simulink model "model"  (R2021a)
settings: Solver=VariableStepAuto  StartTime=0.0  StopTime=20  FixedStep=1/2000  RelTol=1e-3
undefined symbols (not defined in the file or in its folder): DiscIntNeverNeededParam, F, F_I, g, K_lqr, Kf, L, l_p, l_rod, l_t, Local, m_c, m_p, m_wa, PendController, saturationVal, sys_ss, Ts, X, Y, Z
libraries: sm_lib x38, nesl_utility x8, pid_lib x4, sm_cable_examples_lib x4, simulink x2
(part 1 of 2)
settings Model: Creator=tmp  LastModifiedBy=jonas
settings DebuggingCC: SFMachineParentedDataDiag=warning

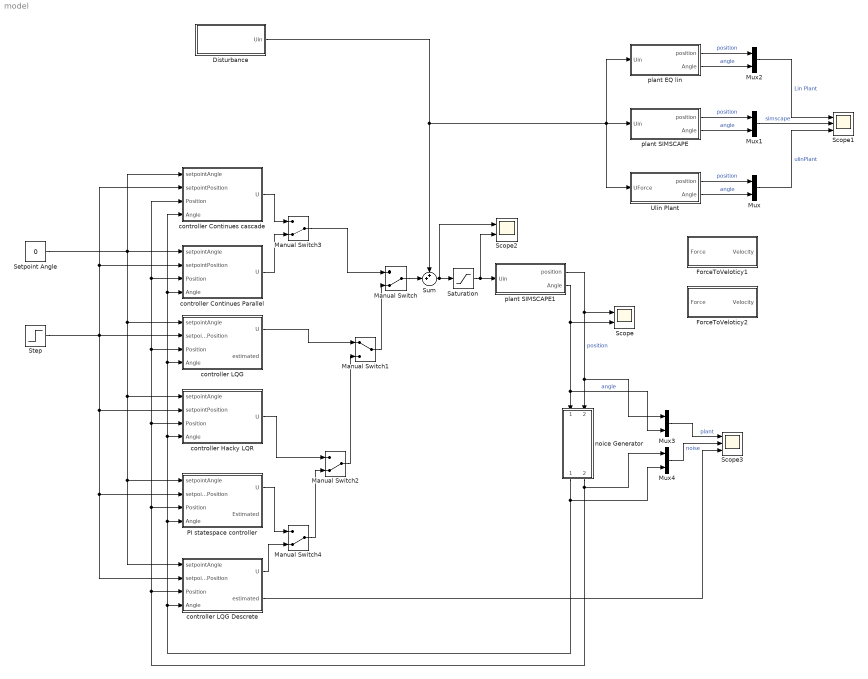
== system model ==
  Disturbance : Subsystem
  ForceToVeloticy1 : Subsystem
  ForceToVeloticy2 : Subsystem
  Manual Switch{,2..4} (4 alike) : ManualSwitch  CurrentSetting=0
  Manual Switch1 : ManualSwitch
  Mux{,1..4} (5 alike) : Mux  Inputs=2
  PI statespace controller : Subsystem
  Saturation : Saturate  UpperLimit=saturationVal  LowerLimit=-saturationVal
  Scope : Scope  NumInputPorts=2
  Scope1 : Scope  NumInputPorts=3
  Scope2 : Scope  NumInputPorts=2
  Scope3 : Scope  NumInputPorts=3
  Setpoint Angle : Constant  Value=0
  Step : Step  Time=5  After=0.5  SampleTime=0
  Sum : Sum  Inputs=++|
  Ulin Plant : Subsystem
  controller Continues Parallel : Subsystem
  controller Continues cascade : Subsystem
  controller Hacky LQR : Subsystem
  controller LQG : Subsystem
  controller LQG Descrete : Subsystem
  noice Generator : Subsystem
  plant EQ lin : Subsystem
  plant SIMSCAPE : Subsystem
  plant SIMSCAPE1 : Subsystem
  wires:
  plant SIMSCAPE1/1(position) -> Mux3/1, noice Generator/2(position), Scope/1  "position"
  plant SIMSCAPE1/2(Angle) -> Mux3/2, noice Generator/1(angle), Scope/2  "angle"
  Step/1 -> controller LQG Descrete/2(setpointPosition), PI statespace controller/2(setpointPosition), controller Hacky LQR/2(setpointPosition), controller LQG/2(setpointPosition), controller Continues cascade/2(setpointPosition), controller Continues Parallel/2(setpointPosition)
  Setpoint Angle/1 -> controller Continues cascade/1(setpointAngle), controller LQG/1(setpointAngle), controller LQG Descrete/1(setpointAngle), PI statespace controller/1(setpointAngle), controller Hacky LQR/1(setpointAngle), controller Continues Parallel/1(setpointAngle)
  Manual Switch3/1 -> Manual Switch/1
  controller Continues Parallel/1(U) -> Manual Switch3/2
  controller Continues cascade/1(U) -> Manual Switch3/1
  Sum/1 -> Saturation/1, Scope2/1
  Ulin Plant/1(position) -> Mux/1  "position"
  Ulin Plant/2(Angle) -> Mux/2  "angle"
  plant SIMSCAPE/1(position) -> Mux1/1  "position"
  plant SIMSCAPE/2(Angle) -> Mux1/2  "angle"
  Mux/1 -> Scope1/3  "ulinPlant"
  Mux1/1 -> Scope1/2  "simscape"
  Disturbance/1(Uin) -> Sum/1, Ulin Plant/1(UForce), plant EQ lin/1(Uin), plant SIMSCAPE/1(Uin)
  Manual Switch/1 -> Sum/2
  plant EQ lin/2(Angle) -> Mux2/2  "angle"
  plant EQ lin/1(position) -> Mux2/1  "position"
  Mux2/1 -> Scope1/1  "Lin Plant"
  controller LQG/1(U) -> Manual Switch1/1
  Manual Switch1/1 -> Manual Switch/2
  Manual Switch2/1 -> Manual Switch1/2
  controller Hacky LQR/1(U) -> Manual Switch2/1
  noice Generator/1(angleOut) -> Mux4/2, controller LQG Descrete/4(Angle), controller Continues cascade/4(Angle), controller Continues Parallel/4(Angle), controller LQG/4(Angle), controller Hacky LQR/4(Angle), PI statespace controller/4(Angle)
  noice Generator/2(positionOut) -> Mux4/1, controller Continues cascade/3(Position), controller Continues Parallel/3(Position), controller LQG/3(Position), controller Hacky LQR/3(Position), PI statespace controller/3(Position), controller LQG Descrete/3(Position)
  Mux3/1 -> Scope3/1  "plant"
  Mux4/1 -> Scope3/2  "noise"
  Saturation/1 -> plant SIMSCAPE1/1(Uin), Scope2/2
  controller LQG Descrete/1(U) -> Manual Switch4/2
  PI statespace controller/1(U) -> Manual Switch4/1
  Manual Switch4/1 -> Manual Switch2/2
  controller LQG Descrete/2(estimated) -> Scope3/3

== system model/Disturbance ==
  Gain1 : Gain
  Step2 : Step  SampleTime=0
  Step3 : Step  Time=1.1  After=-1  SampleTime=0
  Step4 : Step  Time=4  After=-0.5  SampleTime=0
  Step5 : Step  Time=4.1  After=0.5  SampleTime=0
  Sum3 : Sum  Inputs=++++
  Uin : Outport
  wires:
  Step5/1 -> Sum3/4
  Sum3/1 -> Gain1/1
  Step4/1 -> Sum3/3
  Gain1/1 -> Uin/1
  Step3/1 -> Sum3/2
  Step2/1 -> Sum3/1

== system model/ForceToVeloticy1 ==
  Force : Inport
  Gain : Gain  Gain=1/m_c
  Integrator : Integrator
  Velocity : Outport
  wires:
  Force/1 -> Gain/1
  Gain/1 -> Integrator/1
  Integrator/1 -> Velocity/1

== system model/ForceToVeloticy2 ==
  Force : Inport
  Gain : Gain  Gain=1/m_c
  Integrator : Integrator
  Velocity : Outport
  wires:
  Force/1 -> Gain/1
  Gain/1 -> Integrator/1
  Integrator/1 -> Velocity/1

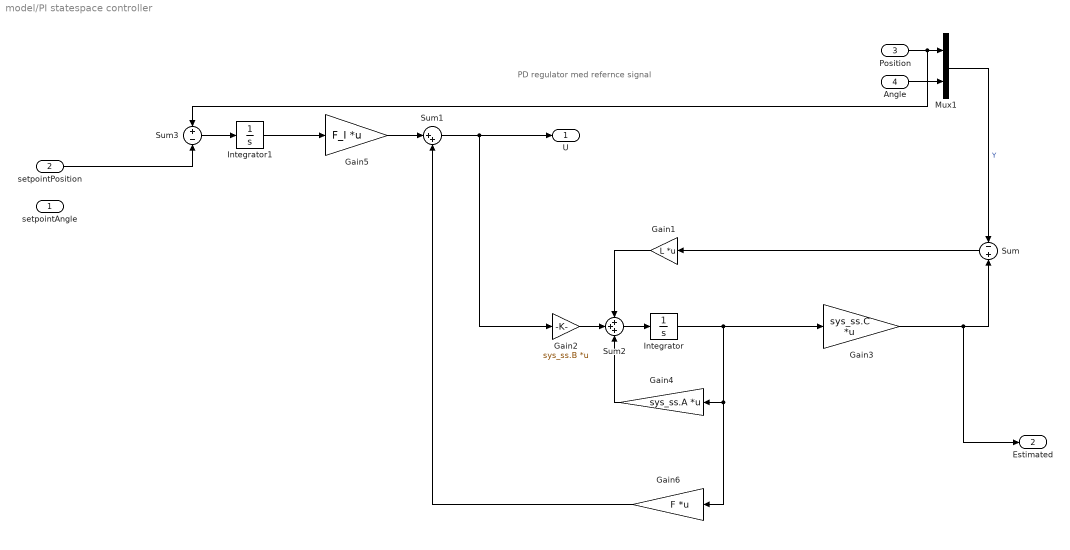
== system model/PI statespace controller ==
  note: PD regulator med refernce signal
  setpointAngle : Inport
  setpointPosition : Inport  Port=2
  Position : Inport  Port=3
  Angle : Inport  Port=4
  Gain1 : Gain  Gain=L  Multiplication=Matrix(K*u)
  Gain2 : Gain  Gain=sys_ss.B  Multiplication=Matrix(K*u)
  Gain3 : Gain  Gain=sys_ss.C  Multiplication=Matrix(K*u)
  Gain4 : Gain  Gain=sys_ss.A  Multiplication=Matrix(K*u)
  Gain5 : Gain  Gain=F_I  Multiplication=Matrix(K*u)
  Gain6 : Gain  Gain=F  Multiplication=Matrix(K*u)
  Integrator : Integrator  IgnoreLimit=on
  Integrator1 : Integrator
  Mux1 : Mux  Inputs=2
  Sum : Sum  Inputs=-+
  Sum1 : Sum  Inputs=|++
  Sum2 : Sum  Inputs=+++
  Sum3 : Sum  Inputs=+-
  U : Outport
  Estimated : Outport  Port=2
  wires:
  Angle/1 -> Mux1/2
  Position/1 -> Sum3/1, Mux1/1
  Gain1/1 -> Sum2/1
  Gain2/1 -> Sum2/2
  Gain3/1 -> Estimated/1, Sum/2
  Integrator/1 -> Gain6/1, Gain4/1, Gain3/1
  Gain4/1 -> Sum2/3
  Sum2/1 -> Integrator/1
  Sum/1 -> Gain1/1
  Mux1/1 -> Sum/1  "Y"
  Sum1/1 -> Gain2/1, U/1
  Gain5/1 -> Sum1/1
  Integrator1/1 -> Gain5/1
  Sum3/1 -> Integrator1/1
  Gain6/1 -> Sum1/2
  setpointPosition/1 -> Sum3/2

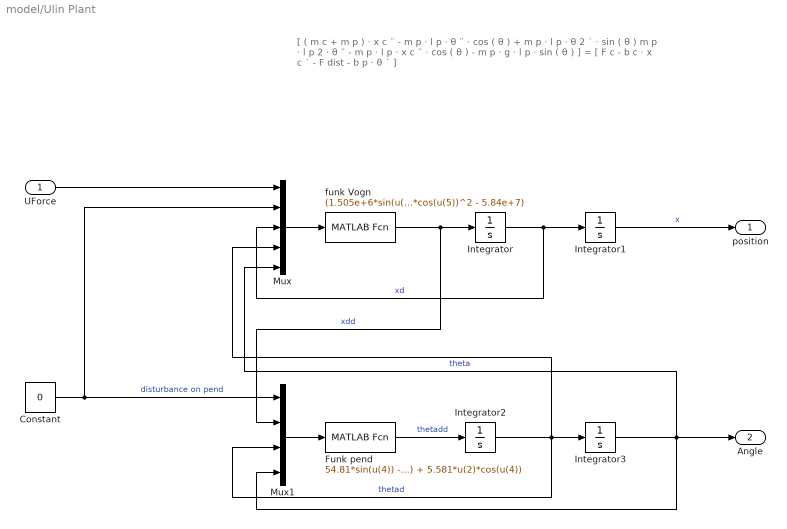
== system model/Ulin Plant ==
  note: [ ( m c + m p ) ⋅ x c ¨ - m p ⋅ l p ⋅ θ ¨ ⋅ cos ( θ ) + m p ⋅ l p ⋅ θ 2 ˙ ⋅ sin ( θ ) m p ⋅ l p 2 ⋅ θ ¨ - m p ⋅ l p ⋅ x c ¨ ⋅ cos ( θ ) - m p ⋅ g ⋅ l p ⋅ sin ( θ ) ] = [ F c - b c ⋅ x c ˙ - F dist - b p ⋅ θ ˙ ]
  UForce : Inport
  Constant : Constant  Value=0
  Funk pend : MATLABFcn  MATLABFcn=54.81*sin(u(4)) - 0.445*u(3) - 370.9*u(1) + 5.581*u(2)*cos(u(4))  OutputDimensions=1  Output1D=off
  Integrator{,1..3} (4 alike) : Integrator
  Mux : Mux  Inputs=5
  Mux1 : Mux
  funk Vogn : MATLABFcn  MATLABFcn=(1.505e+6*sin(u(5))*u(4)^2 + 6.697e+5*cos(u(5))*u(4) - 1.0e+8*u(1) + 5.0e+8*u(3) - 8.249e+7*cos(u(5))*sin(u(5)) + 5.582e+8*u(2)*cos(u(5)))/(8.4e+6*cos(u(5))^2 - 5.84e+7)  OutputDimensions=1  Output1D=off
  position : Outport
  Angle : Outport  Port=2
  wires:
  funk Vogn/1 -> Mux1/2, Integrator/1  "xdd"
  Mux/1 -> funk Vogn/1
  Integrator/1 -> Mux/3, Integrator1/1  "xd"
  Integrator1/1 -> position/1  "x"
  Integrator2/1 -> Mux/4, Mux1/3, Integrator3/1  "thetad"
  Funk pend/1 -> Integrator2/1  "thetadd"
  Mux1/1 -> Funk pend/1
  Integrator3/1 -> Mux/5, Mux1/4, Angle/1  "theta"
  UForce/1 -> Mux/1
  Constant/1 -> Mux1/1, Mux/2  "disturbance on pend"

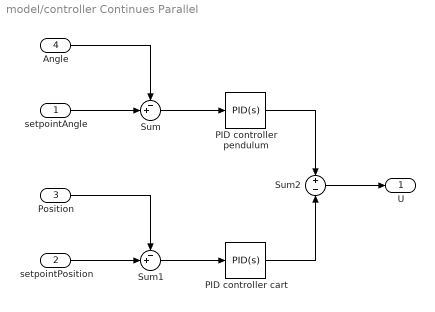
== system model/controller Continues Parallel ==
  setpointAngle : Inport
  setpointPosition : Inport  Port=2
  Position : Inport  Port=3
  Angle : Inport  Port=4
  PID controller cart : pid_lib/PID Controller  Controller=PID  Form=Parallel  TimeDomain=Continuous-time  UseExternalTs=off  SampleTime=-1  IntegratorMethod=Trapezoidal  FilterMethod=Forward Euler  ControllerParametersSource=internal  P=288.854597591641  I=22.5795684687671  D=-65.7392485263013  UseFilter=on  N=4.39394431891132  TunerSelectOption=Transfer Function Based (PID Tuner App)  InitialConditionSource=internal  InitialConditionForIntegrator=0  InitialConditionForFilter=0  DifferentiatorICPrevScaledInput=0  ExternalReset=none  TrackingMode=off  Kt=1  LimitOutput=off  SatLimitsSource=internal  UpperSaturationLimit=inf  LowerSaturationLimit=-inf  LinearizeAsGain=on  AntiWindupMode=none  Kb=1  POutMin=[]  POutMax=[]  IOutMin=[]  IOutMax=[]  DOutMin=[]  DOutMax=[]  NOutMin=[]  NOutMax=[]  SumOutMin=[]  SumOutMax=[]  SaturationOutMin=[]  SaturationOutMax=[]  PParamMin=[]  PParamMax=[]  IParamMin=[]  IParamMax=[]  DParamMin=[]  DParamMax=[]  NParamMin=[]  NParamMax=[]  KbParamMin=[]  KbParamMax=[]  KtParamMin=[]  KtParamMax=[]  KbOutMin=[]  KbOutMax=[]  KtOutMin=[]  KtOutMax=[]  IntegratorOutMin=[]  IntegratorOutMax=[]  FilterOutMin=[]  FilterOutMax=[]  SumI1OutMin=[]  SumI1OutMax=[]  SumI2OutMin=[]  SumI2OutMax=[]  SumI3OutMin=[]  SumI3OutMax=[]  SumI4OutMin=[]  SumI4OutMax=[]  SumDOutMin=[]  SumDOutMax=[]  DifferentiatorOutMin=[]  DifferentiatorOutMax=[]  FilterDiffOutCoefMin=[]  FilterDiffOutCoefMax=[]  ReciprocalOutMin=[]  ReciprocalOutMax=[]  SumDenOutMin=[]  SumDenOutMax=[]  SumNumOutMin=[]  SumNumOutMax=[]  DivideOutMin=[]  DivideOutMax=[]  UdiffTsProdOutMin=[]  UdiffTsProdOutMax=[]  NTsProdOutMin=[]  NTsProdOutMax=[]  UintegralTsProdOutMin=[]  UintegralTsProdOutMax=[]  UngainTsProdOutMin=[]  UngainTsProdOutMax=[]  IntegratorContinuousStateAttributes=''  IntegratorStateMustResolveToSignalObject=off  IntegratorRTWStateStorageClass=Auto  FilterContinuousStateAttributes=''  FilterStateMustResolveToSignalObject=off  FilterRTWStateStorageClass=Auto  ParallelPVariant=InternalParameters  IdealPVariant=Disabled  IVariant=InternalParameters  DVariant=InternalParameters  IntegratorVariant=Continuous  SatVariant=Disabled  AWVariant=Passthrough  PCopyVariant=Disabled  TRVariant=Disabled  FdbkBlocksVariant=Forward  IdealPFdbkVariant=Disabled  SatFdbkVariant=Disabled  DerivativeFilterVariant=ContFilter  NVariant=InternalParameters  NCopyVariant=Disabled  FilterICVariant=InternalICsFilter  IntegratorICVariant=InternalICs  ExternalResetVariant=Disabled  TRSumVariant=Passthrough  SumFdbkVariant=Disabled  SumVariant=Sum_PID  TsampFilterVariant=InternalTs  TsampNgainVariant=Passthrough  TsampIntegralVariant=Passthrough  ExternalSaturationOutDataTypeStr=Inherit: Same as second input
  PID controller pendulum : pid_lib/PID Controller  Controller=PID  Form=Parallel  TimeDomain=Continuous-time  UseExternalTs=off  SampleTime=-1  IntegratorMethod=Trapezoidal  FilterMethod=Trapezoidal  ControllerParametersSource=internal  P=PendController.Kp  I=PendController.Ki  D=PendController.Kd  UseFilter=on  N=PendController.Tf  TunerSelectOption=Transfer Function Based (PID Tuner App)  InitialConditionSource=internal  InitialConditionForIntegrator=0  InitialConditionForFilter=0  DifferentiatorICPrevScaledInput=0  ExternalReset=none  TrackingMode=off  Kt=1  LimitOutput=off  SatLimitsSource=internal  UpperSaturationLimit=inf  LowerSaturationLimit=-inf  LinearizeAsGain=on  AntiWindupMode=none  Kb=1  POutMin=[]  POutMax=[]  IOutMin=[]  IOutMax=[]  DOutMin=[]  DOutMax=[]  NOutMin=[]  NOutMax=[]  SumOutMin=[]  SumOutMax=[]  SaturationOutMin=[]  SaturationOutMax=[]  PParamMin=[]  PParamMax=[]  IParamMin=[]  IParamMax=[]  DParamMin=[]  DParamMax=[]  NParamMin=[]  NParamMax=[]  KbParamMin=[]  KbParamMax=[]  KtParamMin=[]  KtParamMax=[]  KbOutMin=[]  KbOutMax=[]  KtOutMin=[]  KtOutMax=[]  IntegratorOutMin=[]  IntegratorOutMax=[]  FilterOutMin=[]  FilterOutMax=[]  SumI1OutMin=[]  SumI1OutMax=[]  SumI2OutMin=[]  SumI2OutMax=[]  SumI3OutMin=[]  SumI3OutMax=[]  SumI4OutMin=[]  SumI4OutMax=[]  SumDOutMin=[]  SumDOutMax=[]  DifferentiatorOutMin=[]  DifferentiatorOutMax=[]  FilterDiffOutCoefMin=[]  FilterDiffOutCoefMax=[]  ReciprocalOutMin=[]  ReciprocalOutMax=[]  SumDenOutMin=[]  SumDenOutMax=[]  SumNumOutMin=[]  SumNumOutMax=[]  DivideOutMin=[]  DivideOutMax=[]  UdiffTsProdOutMin=[]  UdiffTsProdOutMax=[]  NTsProdOutMin=[]  NTsProdOutMax=[]  UintegralTsProdOutMin=[]  UintegralTsProdOutMax=[]  UngainTsProdOutMin=[]  UngainTsProdOutMax=[]  IntegratorContinuousStateAttributes=''  IntegratorStateMustResolveToSignalObject=off  IntegratorRTWStateStorageClass=Auto  FilterContinuousStateAttributes=''  FilterStateMustResolveToSignalObject=off  FilterRTWStateStorageClass=Auto  ParallelPVariant=InternalParameters  IdealPVariant=Disabled  IVariant=InternalParameters  DVariant=InternalParameters  IntegratorVariant=Continuous  SatVariant=Disabled  AWVariant=Passthrough  PCopyVariant=Disabled  TRVariant=Disabled  FdbkBlocksVariant=Forward  IdealPFdbkVariant=Disabled  SatFdbkVariant=Disabled  DerivativeFilterVariant=ContFilter  NVariant=InternalParameters  NCopyVariant=Disabled  FilterICVariant=InternalICsFilter  IntegratorICVariant=InternalICs  ExternalResetVariant=Disabled  TRSumVariant=Passthrough  SumFdbkVariant=Disabled  SumVariant=Sum_PID  TsampFilterVariant=InternalTs  TsampNgainVariant=Passthrough  TsampIntegralVariant=Passthrough  ExternalSaturationOutDataTypeStr=Inherit: Same as second input
  Sum : Sum  Inputs=-+|
  Sum1 : Sum  Inputs=-+|
  Sum2 : Sum  Inputs=+-
  U : Outport
  wires:
  setpointAngle/1 -> Sum/2
  setpointPosition/1 -> Sum1/2
  Sum1/1 -> PID controller cart/1
  Angle/1 -> Sum/1
  Position/1 -> Sum1/1
  Sum2/1 -> U/1
  PID controller pendulum/1 -> Sum2/1
  Sum/1 -> PID controller pendulum/1
  PID controller cart/1 -> Sum2/2

== system model/controller Continues cascade ==
  setpointAngle : Inport
  setpointPosition : Inport  Port=2
  Position : Inport  Port=3
  Angle : Inport  Port=4
  PID controller cart : pid_lib/PID Controller  Controller=PID  Form=Parallel  TimeDomain=Continuous-time  UseExternalTs=off  SampleTime=-1  IntegratorMethod=Trapezoidal  FilterMethod=Forward Euler  ControllerParametersSource=internal  P=-0.000734383045978884  I=-1.95673604455145e-06  D=-0.0382887909261764  UseFilter=on  N=0.989806605756417  TunerSelectOption=Transfer Function Based (PID Tuner App)  InitialConditionSource=internal  InitialConditionForIntegrator=0  InitialConditionForFilter=0  DifferentiatorICPrevScaledInput=0  ExternalReset=none  TrackingMode=off  Kt=1  LimitOutput=off  SatLimitsSource=internal  UpperSaturationLimit=inf  LowerSaturationLimit=-inf  LinearizeAsGain=on  AntiWindupMode=none  Kb=1  POutMin=[]  POutMax=[]  IOutMin=[]  IOutMax=[]  DOutMin=[]  DOutMax=[]  NOutMin=[]  NOutMax=[]  SumOutMin=[]  SumOutMax=[]  SaturationOutMin=[]  SaturationOutMax=[]  PParamMin=[]  PParamMax=[]  IParamMin=[]  IParamMax=[]  DParamMin=[]  DParamMax=[]  NParamMin=[]  NParamMax=[]  KbParamMin=[]  KbParamMax=[]  KtParamMin=[]  KtParamMax=[]  KbOutMin=[]  KbOutMax=[]  KtOutMin=[]  KtOutMax=[]  IntegratorOutMin=[]  IntegratorOutMax=[]  FilterOutMin=[]  FilterOutMax=[]  SumI1OutMin=[]  SumI1OutMax=[]  SumI2OutMin=[]  SumI2OutMax=[]  SumI3OutMin=[]  SumI3OutMax=[]  SumI4OutMin=[]  SumI4OutMax=[]  SumDOutMin=[]  SumDOutMax=[]  DifferentiatorOutMin=[]  DifferentiatorOutMax=[]  FilterDiffOutCoefMin=[]  FilterDiffOutCoefMax=[]  ReciprocalOutMin=[]  ReciprocalOutMax=[]  SumDenOutMin=[]  SumDenOutMax=[]  SumNumOutMin=[]  SumNumOutMax=[]  DivideOutMin=[]  DivideOutMax=[]  UdiffTsProdOutMin=[]  UdiffTsProdOutMax=[]  NTsProdOutMin=[]  NTsProdOutMax=[]  UintegralTsProdOutMin=[]  UintegralTsProdOutMax=[]  UngainTsProdOutMin=[]  UngainTsProdOutMax=[]  IntegratorContinuousStateAttributes=''  IntegratorStateMustResolveToSignalObject=off  IntegratorRTWStateStorageClass=Auto  FilterContinuousStateAttributes=''  FilterStateMustResolveToSignalObject=off  FilterRTWStateStorageClass=Auto  ParallelPVariant=InternalParameters  IdealPVariant=Disabled  IVariant=InternalParameters  DVariant=InternalParameters  IntegratorVariant=Continuous  SatVariant=Disabled  AWVariant=Passthrough  PCopyVariant=Disabled  TRVariant=Disabled  FdbkBlocksVariant=Forward  IdealPFdbkVariant=Disabled  SatFdbkVariant=Disabled  DerivativeFilterVariant=ContFilter  NVariant=InternalParameters  NCopyVariant=Disabled  FilterICVariant=InternalICsFilter  IntegratorICVariant=InternalICs  ExternalResetVariant=Disabled  TRSumVariant=Passthrough  SumFdbkVariant=Disabled  SumVariant=Sum_PID  TsampFilterVariant=InternalTs  TsampNgainVariant=Passthrough  TsampIntegralVariant=Passthrough  ExternalSaturationOutDataTypeStr=Inherit: Same as second input
  PID controller pendulum : pid_lib/PID Controller  Controller=PID  Form=Parallel  TimeDomain=Continuous-time  UseExternalTs=off  SampleTime=-1  IntegratorMethod=Trapezoidal  FilterMethod=Trapezoidal  ControllerParametersSource=internal  P=PendController.Kp  I=PendController.Ki  D=PendController.Kd  UseFilter=on  N=PendController.Tf  TunerSelectOption=Transfer Function Based (PID Tuner App)  InitialConditionSource=internal  InitialConditionForIntegrator=0  InitialConditionForFilter=0  DifferentiatorICPrevScaledInput=0  ExternalReset=none  TrackingMode=off  Kt=1  LimitOutput=off  SatLimitsSource=internal  UpperSaturationLimit=inf  LowerSaturationLimit=-inf  LinearizeAsGain=on  AntiWindupMode=none  Kb=1  POutMin=[]  POutMax=[]  IOutMin=[]  IOutMax=[]  DOutMin=[]  DOutMax=[]  NOutMin=[]  NOutMax=[]  SumOutMin=[]  SumOutMax=[]  SaturationOutMin=[]  SaturationOutMax=[]  PParamMin=[]  PParamMax=[]  IParamMin=[]  IParamMax=[]  DParamMin=[]  DParamMax=[]  NParamMin=[]  NParamMax=[]  KbParamMin=[]  KbParamMax=[]  KtParamMin=[]  KtParamMax=[]  KbOutMin=[]  KbOutMax=[]  KtOutMin=[]  KtOutMax=[]  IntegratorOutMin=[]  IntegratorOutMax=[]  FilterOutMin=[]  FilterOutMax=[]  SumI1OutMin=[]  SumI1OutMax=[]  SumI2OutMin=[]  SumI2OutMax=[]  SumI3OutMin=[]  SumI3OutMax=[]  SumI4OutMin=[]  SumI4OutMax=[]  SumDOutMin=[]  SumDOutMax=[]  DifferentiatorOutMin=[]  DifferentiatorOutMax=[]  FilterDiffOutCoefMin=[]  FilterDiffOutCoefMax=[]  ReciprocalOutMin=[]  ReciprocalOutMax=[]  SumDenOutMin=[]  SumDenOutMax=[]  SumNumOutMin=[]  SumNumOutMax=[]  DivideOutMin=[]  DivideOutMax=[]  UdiffTsProdOutMin=[]  UdiffTsProdOutMax=[]  NTsProdOutMin=[]  NTsProdOutMax=[]  UintegralTsProdOutMin=[]  UintegralTsProdOutMax=[]  UngainTsProdOutMin=[]  UngainTsProdOutMax=[]  IntegratorContinuousStateAttributes=''  IntegratorStateMustResolveToSignalObject=off  IntegratorRTWStateStorageClass=Auto  FilterContinuousStateAttributes=''  FilterStateMustResolveToSignalObject=off  FilterRTWStateStorageClass=Auto  ParallelPVariant=InternalParameters  IdealPVariant=Disabled  IVariant=InternalParameters  DVariant=InternalParameters  IntegratorVariant=Continuous  SatVariant=Disabled  AWVariant=Passthrough  PCopyVariant=Disabled  TRVariant=Disabled  FdbkBlocksVariant=Forward  IdealPFdbkVariant=Disabled  SatFdbkVariant=Disabled  DerivativeFilterVariant=ContFilter  NVariant=InternalParameters  NCopyVariant=Disabled  FilterICVariant=InternalICsFilter  IntegratorICVariant=InternalICs  ExternalResetVariant=Disabled  TRSumVariant=Passthrough  SumFdbkVariant=Disabled  SumVariant=Sum_PID  TsampFilterVariant=InternalTs  TsampNgainVariant=Passthrough  TsampIntegralVariant=Passthrough  ExternalSaturationOutDataTypeStr=Inherit: Same as second input
  Sum : Sum  Inputs=-+|
  Sum1 : Sum  Inputs=-+|
  U : Outport
  wires:
  setpointPosition/1 -> Sum1/2
  Sum1/1 -> PID controller cart/1
  Angle/1 -> Sum/1
  Position/1 -> Sum1/1
  PID controller pendulum/1 -> U/1
  Sum/1 -> PID controller pendulum/1
  PID controller cart/1 -> Sum/2

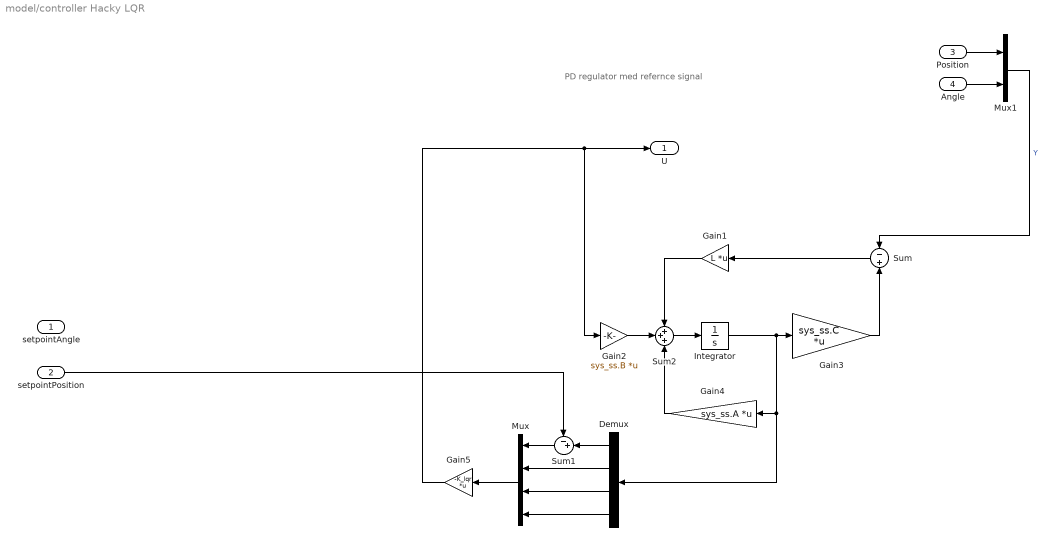
== system model/controller Hacky LQR ==
  note: PD regulator med refernce signal
  setpointAngle : Inport
  setpointPosition : Inport  Port=2
  Position : Inport  Port=3
  Angle : Inport  Port=4
  Demux : Demux
  Gain1 : Gain  Gain=L  Multiplication=Matrix(K*u)
  Gain2 : Gain  Gain=sys_ss.B  Multiplication=Matrix(K*u)
  Gain3 : Gain  Gain=sys_ss.C  Multiplication=Matrix(K*u)
  Gain4 : Gain  Gain=sys_ss.A  Multiplication=Matrix(K*u)
  Gain5 : Gain  Gain=-K_lqr  Multiplication=Matrix(K*u)
  Integrator : Integrator  IgnoreLimit=on
  Mux : Mux
  Mux1 : Mux  Inputs=2
  Sum : Sum  Inputs=-+
  Sum1 : Sum  Inputs=-+|
  Sum2 : Sum  Inputs=+++
  U : Outport
  wires:
  Angle/1 -> Mux1/2
  Position/1 -> Mux1/1
  Gain1/1 -> Sum2/1
  Gain2/1 -> Sum2/2
  Gain3/1 -> Sum/2
  Integrator/1 -> Demux/1, Gain4/1, Gain3/1
  Gain4/1 -> Sum2/3
  Sum2/1 -> Integrator/1
  Sum/1 -> Gain1/1
  Mux1/1 -> Sum/1  "Y"
  Mux/1 -> Gain5/1
  Demux/2 -> Mux/2
  Demux/3 -> Mux/3
  Demux/4 -> Mux/4
  Sum1/1 -> Mux/1
  Demux/1 -> Sum1/2
  setpointPosition/1 -> Sum1/1
  Gain5/1 -> Gain2/1, U/1

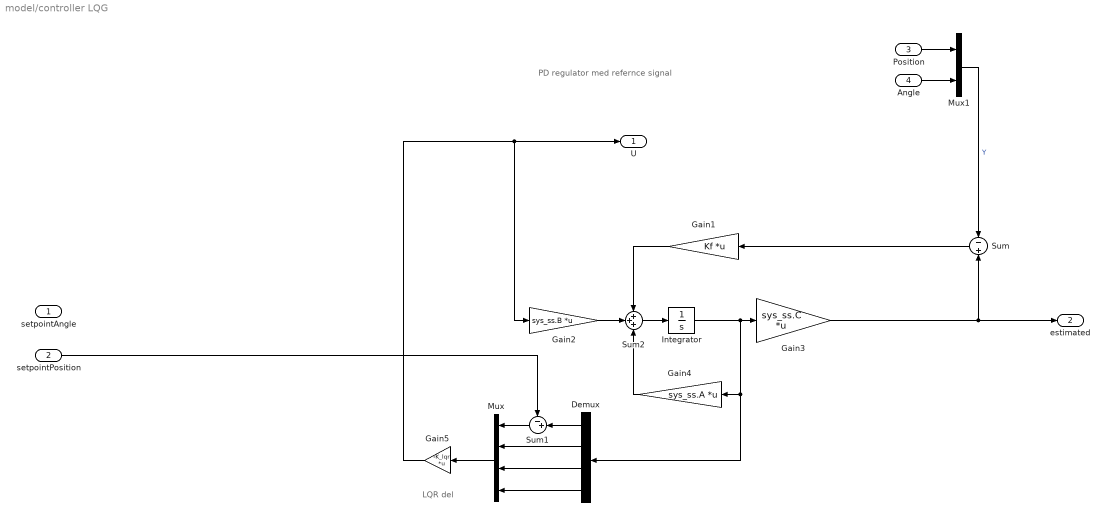
== system model/controller LQG ==
  note: LQR del
  note: PD regulator med refernce signal
  setpointAngle : Inport
  setpointPosition : Inport  Port=2
  Position : Inport  Port=3
  Angle : Inport  Port=4
  Demux : Demux
  Gain1 : Gain  Gain=Kf  Multiplication=Matrix(K*u)
  Gain2 : Gain  Gain=sys_ss.B  Multiplication=Matrix(K*u)
  Gain3 : Gain  Gain=sys_ss.C  Multiplication=Matrix(K*u)
  Gain4 : Gain  Gain=sys_ss.A  Multiplication=Matrix(K*u)
  Gain5 : Gain  Gain=-K_lqr  Multiplication=Matrix(K*u)
  Integrator : Integrator  IgnoreLimit=on
  Mux : Mux
  Mux1 : Mux  Inputs=2
  Sum : Sum  Inputs=-+
  Sum1 : Sum  Inputs=-+|
  Sum2 : Sum  Inputs=+++
  U : Outport
  estimated : Outport  Port=2
  wires:
  Angle/1 -> Mux1/2
  Position/1 -> Mux1/1
  Gain1/1 -> Sum2/1
  Gain2/1 -> Sum2/2
  Gain3/1 -> estimated/1, Sum/2
  Gain4/1 -> Sum2/3
  Sum2/1 -> Integrator/1
  Sum/1 -> Gain1/1
  Mux1/1 -> Sum/1  "Y"
  Mux/1 -> Gain5/1
  Demux/2 -> Mux/2
  Demux/3 -> Mux/3
  Demux/4 -> Mux/4
  Sum1/1 -> Mux/1
  Demux/1 -> Sum1/2
  setpointPosition/1 -> Sum1/1
  Gain5/1 -> U/1, Gain2/1
  Integrator/1 -> Demux/1, Gain4/1, Gain3/1

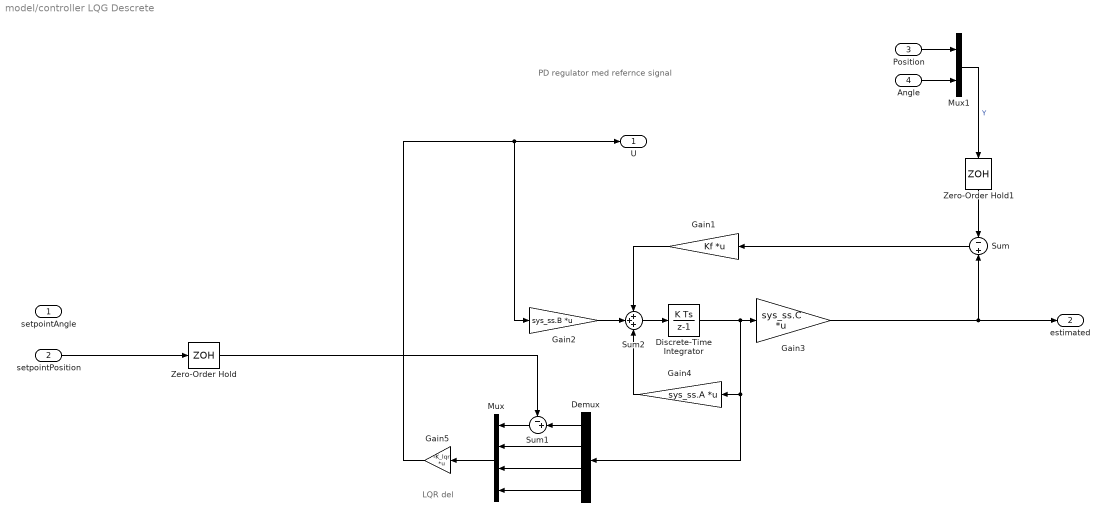
== system model/controller LQG Descrete ==
  note: LQR del
  note: PD regulator med refernce signal
  setpointAngle : Inport
  setpointPosition : Inport  Port=2
  Position : Inport  Port=3
  Angle : Inport  Port=4
  Demux : Demux
  Discrete-Time Integrator : DiscreteIntegrator  SampleTime=Ts  ICPrevOutput=DiscIntNeverNeededParam  ICPrevScaledInput=DiscIntNeverNeededParam
  Gain1 : Gain  Gain=Kf  Multiplication=Matrix(K*u)
  Gain2 : Gain  Gain=sys_ss.B  Multiplication=Matrix(K*u)
  Gain3 : Gain  Gain=sys_ss.C  Multiplication=Matrix(K*u)
  Gain4 : Gain  Gain=sys_ss.A  Multiplication=Matrix(K*u)
  Gain5 : Gain  Gain=-K_lqr  Multiplication=Matrix(K*u)
  Mux : Mux
  Mux1 : Mux  Inputs=2
  Sum : Sum  Inputs=-+
  Sum1 : Sum  Inputs=-+|
  Sum2 : Sum  Inputs=+++
  Zero-Order Hold : ZeroOrderHold  SampleTime=Ts
  Zero-Order Hold1 : ZeroOrderHold  SampleTime=Ts
  U : Outport
  estimated : Outport  Port=2
  wires:
  Angle/1 -> Mux1/2
  Position/1 -> Mux1/1
  Gain1/1 -> Sum2/1
  Gain2/1 -> Sum2/2
  Gain3/1 -> estimated/1, Sum/2
  Gain4/1 -> Sum2/3
  Sum2/1 -> Discrete-Time Integrator/1
  Sum/1 -> Gain1/1
  Mux1/1 -> Zero-Order Hold1/1  "Y"
  Mux/1 -> Gain5/1
  Demux/2 -> Mux/2
  Demux/3 -> Mux/3
  Demux/4 -> Mux/4
  Sum1/1 -> Mux/1
  Demux/1 -> Sum1/2
  setpointPosition/1 -> Zero-Order Hold/1
  Gain5/1 -> U/1, Gain2/1
  Discrete-Time Integrator/1 -> Demux/1, Gain4/1, Gain3/1
  Zero-Order Hold/1 -> Sum1/1
  Zero-Order Hold1/1 -> Sum/1

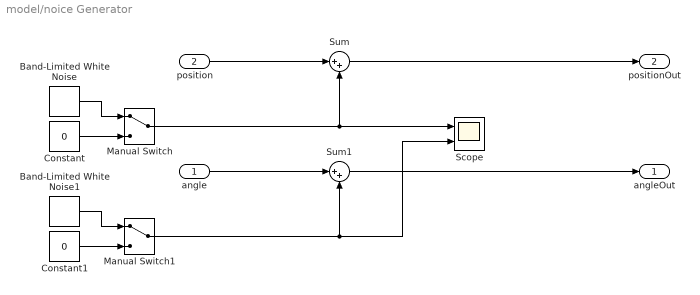
== system model/noice Generator ==
  angle : Inport
  position : Inport  Port=2
  Band-Limited White Noise : simulink/Sources/Band-Limited White Noise  Cov=[0.0000001]  Ts=0.01  seed=[23341]
  Band-Limited White Noise1 : simulink/Sources/Band-Limited White Noise  Cov=[0.0000001]  Ts=0.01  seed=[10000]
  Constant : Constant  Value=0
  Constant1 : Constant  Value=0
  Manual Switch : ManualSwitch
  Manual Switch1 : ManualSwitch
  Scope : Scope  NumInputPorts=2
  Sum : Sum  Inputs=|++
  Sum1 : Sum  Inputs=|++
  angleOut : Outport
  positionOut : Outport  Port=2
  wires:
  position/1 -> Sum/1
  Sum/1 -> positionOut/1
  Sum1/1 -> angleOut/1
  angle/1 -> Sum1/1
  Band-Limited White Noise/1 -> Manual Switch/1
  Constant/1 -> Manual Switch/2
  Constant1/1 -> Manual Switch1/2
  Band-Limited White Noise1/1 -> Manual Switch1/1
  Manual Switch1/1 -> Sum1/2, Scope/2
  Manual Switch/1 -> Sum/2, Scope/1

== system model/plant EQ lin ==
  Uin : Inport
  Demux : Demux
  State-Space : StateSpace  A=sys_ss.A  B=sys_ss.B  C=eye(4)  D=[0;0;0;0]  InitialCondition=0
  position : Outport
  Angle : Outport  Port=2
  wires:
  Uin/1 -> State-Space/1
  Demux/3 -> Angle/1
  State-Space/1 -> Demux/1
  Demux/1 -> position/1

== system model/plant SIMSCAPE ==
  Uin : Inport
  Base : Subsystem
  Configuration : Subsystem
  PS-Simulink Converter : nesl_utility/PS-Simulink Converter  PhysicalDomain=network_engine_domain  SubClassName=ps_output  LeftPortType=input  RightPortType=output  PseudoPeriodic=off  Frequencies=[]  Unit=inherit  AffineConversion=off
      settings: SourceProductBaseCode=PW,SS
  PS-Simulink Converter1 : nesl_utility/PS-Simulink Converter  PhysicalDomain=network_engine_domain  SubClassName=ps_output  LeftPortType=input  RightPortType=output  PseudoPeriodic=off  Frequencies=[]  Unit=inherit  AffineConversion=off
      settings: SourceProductBaseCode=PW,SS
  Plant : Subsystem
      settings: PortSchema="{\"entries\":[{\"content\":{\"sides\":[{\"content\":{\"connectorIds\":[\"LConn1\",\"In1\",\"LConn2\",\"LConn3\"]},\"type\":\"ConnectorPlacement.EquallySpacedRectSide\",\"uuid\":\"e241dd80-f9a1-4c3d-bd3c-4b3bd119c000\"},{\"content\":{\"connectorIds\":[],\"side\":\"RIGHT\"},\"type\":\"ConnectorPlacement.EquallySpacedRectSide\",\"uuid\":\"50ff246f-1c39-4ae1-b10f-6d3ede22cdb7\"},{\"content\":{\"connectorIds\":[],\"side\":\"TOP\"},\"type\":\"ConnectorPlacement.EquallySpacedRectSide\",\"uuid\":\"3277ae83-9f73-4616-bf6d-fc59e06ded2c\"}]},\"type\":\"ConnectorPlacement.EquallySpacedConnector\",\"uuid\":\"16b9ee55-2353-4e36-979f-af01577ad86e\"}],\"packageUris\":[\"http://schema.mathworks.com/mf0/Connector/R2020b\"],\"version\":\"1.0\"}"
  position : Outport
  Angle : Outport  Port=2
  wires:
  Uin/1 -> Plant/1(force)
  PS-Simulink Converter/1 -> position/1
  PS-Simulink Converter1/1 -> Angle/1
  connections:
  Base/RConn3 -- Configuration/RConn1 -- Plant/LConn1
  PS-Simulink Converter/LConn1 -- Plant/LConn3
  PS-Simulink Converter1/LConn1 -- Plant/LConn2

== system model/plant SIMSCAPE1 ==
  Uin : Inport
  Base : Subsystem
  Configuration : Subsystem
  PS-Simulink Converter : nesl_utility/PS-Simulink Converter  PhysicalDomain=network_engine_domain  SubClassName=ps_output  LeftPortType=input  RightPortType=output  PseudoPeriodic=off  Frequencies=[]  Unit=inherit  AffineConversion=off
      settings: SourceProductBaseCode=PW,SS
  PS-Simulink Converter1 : nesl_utility/PS-Simulink Converter  PhysicalDomain=network_engine_domain  SubClassName=ps_output  LeftPortType=input  RightPortType=output  PseudoPeriodic=off  Frequencies=[]  Unit=inherit  AffineConversion=off
      settings: SourceProductBaseCode=PW,SS
  Plant : Subsystem
      settings: PortSchema="{\"entries\":[{\"content\":{\"sides\":[{\"content\":{\"connectorIds\":[\"LConn1\",\"In1\",\"LConn2\",\"LConn3\"]},\"type\":\"ConnectorPlacement.EquallySpacedRectSide\",\"uuid\":\"e241dd80-f9a1-4c3d-bd3c-4b3bd119c000\"},{\"content\":{\"connectorIds\":[],\"side\":\"RIGHT\"},\"type\":\"ConnectorPlacement.EquallySpacedRectSide\",\"uuid\":\"50ff246f-1c39-4ae1-b10f-6d3ede22cdb7\"},{\"content\":{\"connectorIds\":[],\"side\":\"TOP\"},\"type\":\"ConnectorPlacement.EquallySpacedRectSide\",\"uuid\":\"3277ae83-9f73-4616-bf6d-fc59e06ded2c\"}]},\"type\":\"ConnectorPlacement.EquallySpacedConnector\",\"uuid\":\"16b9ee55-2353-4e36-979f-af01577ad86e\"}],\"packageUris\":[\"http://schema.mathworks.com/mf0/Connector/R2020b\"],\"version\":\"1.0\"}"
  position : Outport
  Angle : Outport  Port=2
  wires:
  Uin/1 -> Plant/1(force)
  PS-Simulink Converter/1 -> position/1
  PS-Simulink Converter1/1 -> Angle/1
  connections:
  Base/RConn3 -- Configuration/RConn1 -- Plant/LConn1
  PS-Simulink Converter/LConn1 -- Plant/LConn3
  PS-Simulink Converter1/LConn1 -- Plant/LConn2

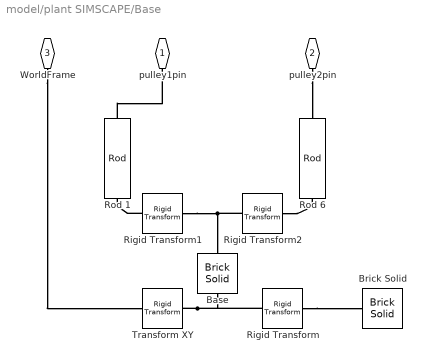
== system model/plant SIMSCAPE/Base ==
  Base : sm_lib/Body Elements/Brick Solid  GraphicAmbientColor=[0.15 0.15 0.15 1.0]  BasedOnType=Density  BrickDimensions=[l_t+0.1 0.02 0.1]  BrickDimensionUnits=m  CenterOfMass=[0 0 0]  CenterOfMassUnits=m  GraphicDiffuseColor=[1.0 1.0 1.0]  Density=1000  DensityUnits=kg/m^3  DoExposeReferenceFrame=off  GraphicEmissiveColor=[0.0 0.0 0.0 1.0]  ExportEntireGeometry=off  SerializedFrames=<Frames><Frame><Id>Frame1</Id><Value><Name>T</Name><Origin><Source>GeometricFeature</Source><FeatureName>+z surface</FeatureName></Origin><PrimaryAxis><DefinedDirection>+Z</DefinedDirection><Source>ReferenceFrame</Source><SourceDirection>+Z</SourceDirection><FeatureName></FeatureName></PrimaryAxis><SecondaryAxis><DefinedDirection>+X</DefinedDirection><Source>ReferenceFrame</Source><SourceDirection>+X</SourceDirection><FeatureName></FeatureName></SecondaryAxis></Value></Frame><Frame><Id>Frame2</Id><Value><Name>B</Name><Origin><Source>GeometricFeature</Source><FeatureName>-z surface</FeatureName></Origin><PrimaryAxis><DefinedDirection>+Z</DefinedDirection><Source>ReferenceFrame</Source><SourceDirection>+Z</SourceDirection><FeatureName></FeatureName></PrimaryAxis><SecondaryAxis><DefinedDirection>+X</DefinedDirection><Source>ReferenceFrame</Source><SourceDirection>+X</SourceDirection><FeatureName></FeatureName></SecondaryAxis></Value></Frame></Frames>  MarkerShape=Sphere  MarkerSize=10  GraphicType=FromGeometry  InertiaType=CalculateFromGeometry  Mass=1  MassUnits=kg  MomentsOfInertia=[1 1 1]  MomentsOfInertiaUnits=kg*m^2  GraphicOpacity=0.75  ProductsOfInertia=[0 0 0]  ProductsOfInertiaUnits=kg*m^2  GraphicShininess=128  GraphicSpecularColor=[0.5 0.5 0.5 1.0]  GraphicVisPropType=SimpleVisualProperties
      settings: SourceProductName=Multibody
  Brick Solid : sm_lib/Body Elements/Brick Solid  GraphicAmbientColor=[0.15 0.15 0.15 1.0]  BasedOnType=Density  BrickDimensions=[l_t 0.05 0.01]  BrickDimensionUnits=m  CenterOfMass=[0 0 0]  CenterOfMassUnits=m  GraphicDiffuseColor=[0.8 0.8 0.8]  Density=1000  DensityUnits=kg/m^3  DoExposeReferenceFrame=on  GraphicEmissiveColor=[0.0 0.0 0.0 1.0]  ExportEntireGeometry=off  SerializedFrames=<Frames/>  MarkerShape=Sphere  MarkerSize=10  GraphicType=FromGeometry  InertiaType=CalculateFromGeometry  Mass=1  MassUnits=kg  MomentsOfInertia=[1 1 1]  MomentsOfInertiaUnits=kg*m^2  GraphicOpacity=1.0  ProductsOfInertia=[0 0 0]  ProductsOfInertiaUnits=kg*m^2  GraphicShininess=75  GraphicSpecularColor=[0.5 0.5 0.5 1.0]  GraphicVisPropType=SimpleVisualProperties
  Rigid Transform : sm_lib/Frames and Transforms/Rigid Transform  TranslationMethod=Cartesian  TranslationStandardOffset=0  TranslationLengthUnit=m  TranslationStandardAxis=+Z  TranslationCartesianOffset=[0 -0.03 0.0825]  TranslationROffset=0  TranslationROffsetUnits=m  TranslationZOffset=0  TranslationZOffsetUnits=m  TranslationThetaOffset=0  TranslationThetaOffsetUnits=deg  RotationMethod=None  RotationAngleUnits=deg  RotationStandardAxis=+Z  RotationAngle=0.0  RotationArbitraryAxis=[0 0 1]  FollAlignAxisA=+X  BaseAlignAxisA=+Y  FollAlignAxisB=+Y  BaseAlignAxisB=+Z  RotationSequenceAxes=FollowerAxes  RotationSequence=XYX  RotationSequenceAngles=[0 0 0]  RotationSequenceAnglesUnits=deg  RotationMatrix=[1 0 0; 0 1 0; 0 0 1]
  Rigid Transform1 : sm_lib/Frames and Transforms/Rigid Transform  TranslationMethod=Cartesian  TranslationStandardOffset=0  TranslationLengthUnit=m  TranslationStandardAxis=+Z  TranslationCartesianOffset=[-l_t/2 0 -0.05]  TranslationROffset=0  TranslationROffsetUnits=m  TranslationZOffset=0  TranslationZOffsetUnits=m  TranslationThetaOffset=0  TranslationThetaOffsetUnits=deg  RotationMethod=StandardAxis  RotationAngleUnits=deg  RotationStandardAxis=+X  RotationAngle=90  RotationArbitraryAxis=[0 0 1]  FollAlignAxisA=+X  BaseAlignAxisA=+Y  FollAlignAxisB=+Y  BaseAlignAxisB=+Z  RotationSequenceAxes=FollowerAxes  RotationSequence=XYX  RotationSequenceAngles=[0 0 0]  RotationSequenceAnglesUnits=deg  RotationMatrix=[1 0 0; 0 1 0; 0 0 1]
  Rigid Transform2 : sm_lib/Frames and Transforms/Rigid Transform  TranslationMethod=Cartesian  TranslationStandardOffset=0  TranslationLengthUnit=m  TranslationStandardAxis=+Z  TranslationCartesianOffset=[l_t/2 0 -0.05]  TranslationROffset=0  TranslationROffsetUnits=m  TranslationZOffset=0  TranslationZOffsetUnits=m  TranslationThetaOffset=0  TranslationThetaOffsetUnits=deg  RotationMethod=StandardAxis  RotationAngleUnits=deg  RotationStandardAxis=+X  RotationAngle=90  RotationArbitraryAxis=[0 0 1]  FollAlignAxisA=+X  BaseAlignAxisA=+Y  FollAlignAxisB=+Y  BaseAlignAxisB=+Z  RotationSequenceAxes=FollowerAxes  RotationSequence=XYX  RotationSequenceAngles=[0 0 0]  RotationSequenceAnglesUnits=deg  RotationMatrix=[1 0 0; 0 1 0; 0 0 1]
  Rod 1 : sm_cable_examples_lib/Basic/Rod  rod_rad=0.01  rod_len=0.05  rod_rho=7000  rod_color=[0.5 0.5 0.5]  popup_zori=Local +Z  popup_markings=None  mark_radius_range=[0.5 1.01]  mark_length_range=1.005  mark_angle_range=30  mark_color=[1 1 1]
      link override Transform F: TranslationStandardOffset=rod_len/4*z_ori
      settings: SourceProductBaseCode=MS
  Rod 6 : sm_cable_examples_lib/Basic/Rod  rod_rad=0.01  rod_len=0.05  rod_rho=7000  rod_color=[0.5 0.5 0.5]  popup_zori=Local +Z  popup_markings=None  mark_radius_range=[0.5 1.01]  mark_length_range=1.005  mark_angle_range=30  mark_color=[1 1 1]
      link override Transform F: TranslationStandardOffset=rod_len/4*z_ori
      settings: SourceProductBaseCode=MS
  Transform XY : sm_lib/Frames and Transforms/Rigid Transform  TranslationMethod=Cartesian  TranslationStandardOffset=0  TranslationLengthUnit=m  TranslationStandardAxis=+Z  TranslationCartesianOffset=[0 0.03 -0.1]  TranslationROffset=0  TranslationROffsetUnits=m  TranslationZOffset=0  TranslationZOffsetUnits=m  TranslationThetaOffset=0  TranslationThetaOffsetUnits=deg  RotationMethod=StandardAxis  RotationAngleUnits=deg  RotationStandardAxis=+Z  RotationAngle=0  RotationArbitraryAxis=[0 0 1]  FollAlignAxisA=+X  BaseAlignAxisA=+Y  FollAlignAxisB=+Y  BaseAlignAxisB=+Z  RotationSequenceAxes=FollowerAxes  RotationSequence=XYX  RotationSequenceAngles=[0 0 0]  RotationSequenceAnglesUnits=deg  RotationMatrix=[1 0 0; 0 1 0; 0 0 1]
      settings: SourceProductName=Multibody
  pulley1pin : PMIOPort  Side=Right
  pulley2pin : PMIOPort  Port=2  Side=Right
  WorldFrame : PMIOPort  Port=3  Side=Right
  connections:
  Rigid Transform2/LConn1 -- Rigid Transform1/LConn1 -- Base/LConn1
  pulley2pin/RConn1 -- Rod 6/RConn1
  Transform XY/RConn1 -- Base/RConn1 -- Rigid Transform/LConn1
  Rigid Transform/RConn1 -- Brick Solid/RConn1
  Rigid Transform2/RConn1 -- Rod 6/LConn1
  WorldFrame/RConn1 -- Transform XY/LConn1
  Rod 1/RConn1 -- pulley1pin/RConn1
  Rigid Transform1/RConn1 -- Rod 1/LConn1

== system model/plant SIMSCAPE/Configuration ==
  Mechanism Configuration : sm_lib/Utilities/Mechanism Configuration  UniformGravity=Constant  GravityVector=[0 0 -g]  GravityVectorUnits=m/s^2  GravityUnits=m/s^2  LinearizationDelta=0.001  JointModeTransitionNonlinearIterations=2
  Solver Configuration : nesl_utility/Solver Configuration  PhysicalDomain=network_engine_domain  SubClassName=solver  LeftPortType=input  RightPortType=generic  Tones=[]  Harmonics=[]  SimulateNoise=off  Profile=off  UseLocalSampling=off  EnableSwitchedLinearOptims=on  FrequencyDomain=off  UseCCode=off  RelTol=0.001  AbsTol=1e-06  MinStep=1e-09  ToWorkspace=off  RevertToSquareIcSolve=off  NumHomotopyIterations=100  PhasorMode=off  PhasorModeNumHarmonics=1  DoDC=off  ResidualTolerance=1e-09  UseLocalSolver=off  LocalSolverChoice=NE_BACKWARD_EULER_ADVANCER  LocalSolverSampleTime=0.001  DoFixedCost=off  MaxNonlinIter=3  MaxModeIter=2  ComputeImpulses=off  ImpulseIterations=2  LinearAlgebra=auto  EquationFormulation=NE_TIME_EF  DelaysMemoryBudget=1024  AutomaticFiltering=on  FilteringTimeConstant=0.001  PartitionStorageMethod=AS_NEEDED  PartitionMemoryBudget=1024  PartitionMethod=ROBUST
      settings: SourceProductBaseCode=PW,SS
  World Frame : sm_lib/Frames and Transforms/World Frame
  solver : PMIOPort  Side=Right
  connections:
  Solver Configuration/RConn1 -- Mechanism Configuration/RConn1 -- World Frame/RConn1 -- solver/RConn1

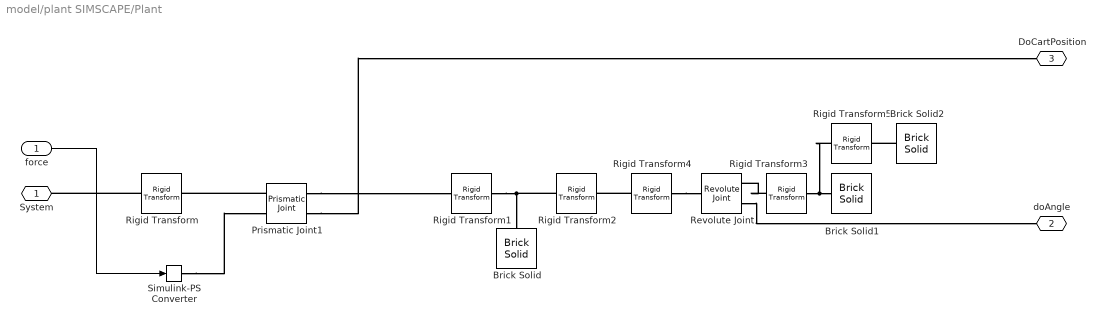
== system model/plant SIMSCAPE/Plant ==
  force : Inport
  Brick Solid : sm_lib/Body Elements/Brick Solid  GraphicAmbientColor=[0.15 0.15 0.15 1.0]  BasedOnType=Mass  BrickDimensions=[0.1 0.025 0.025]  BrickDimensionUnits=m  CenterOfMass=[0 0 0]  CenterOfMassUnits=m  GraphicDiffuseColor=[0.0 0.2 1.0]  Density=1000  DensityUnits=kg/m^3  DoExposeReferenceFrame=on  GraphicEmissiveColor=[0.0 0.0 0.0 1.0]  ExportEntireGeometry=off  SerializedFrames=<Frames/>  MarkerShape=Sphere  MarkerSize=10  GraphicType=FromGeometry  InertiaType=PointMass  Mass=m_c  MassUnits=kg  MomentsOfInertia=[1 1 1]  MomentsOfInertiaUnits=kg*m^2  GraphicOpacity=1.0  ProductsOfInertia=[0 0 0]  ProductsOfInertiaUnits=kg*m^2  GraphicShininess=75  GraphicSpecularColor=[0.5 0.5 0.5 1.0]  GraphicVisPropType=SimpleVisualProperties
  Brick Solid1 : sm_lib/Body Elements/Brick Solid  GraphicAmbientColor=[0.15 0.15 0.15 1.0]  BasedOnType=Mass  BrickDimensions=[l_rod 0.02 0.02]  BrickDimensionUnits=m  CenterOfMass=[0 0 0]  CenterOfMassUnits=m  GraphicDiffuseColor=[1.0 0.0 0.2]  Density=1000  DensityUnits=kg/m^3  DoExposeReferenceFrame=on  GraphicEmissiveColor=[0.0 0.0 0.0 1.0]  ExportEntireGeometry=off  SerializedFrames=<Frames/>  MarkerShape=Sphere  MarkerSize=10  GraphicType=FromGeometry  InertiaType=PointMass  Mass=m_p  MassUnits=kg  MomentsOfInertia=[1 1 1]  MomentsOfInertiaUnits=kg*m^2  GraphicOpacity=1.0  ProductsOfInertia=[0 0 0]  ProductsOfInertiaUnits=kg*m^2  GraphicShininess=75  GraphicSpecularColor=[0.5 0.5 0.5 1.0]  GraphicVisPropType=SimpleVisualProperties
  Brick Solid2 : sm_lib/Body Elements/Brick Solid  GraphicAmbientColor=[0.15 0.15 0.15 1.0]  BasedOnType=Density  BrickDimensions=[0.01 0.01 0.01]  BrickDimensionUnits=m  CenterOfMass=[0 0 0]  CenterOfMassUnits=m  GraphicDiffuseColor=[0.5 0.5 0.5]  Density=1000  DensityUnits=kg/m^3  DoExposeReferenceFrame=on  GraphicEmissiveColor=[0.0 0.0 0.0 1.0]  ExportEntireGeometry=off  SerializedFrames=<Frames/>  MarkerShape=Sphere  MarkerSize=10  GraphicType=FromGeometry  InertiaType=PointMass  Mass=m_wa  MassUnits=kg  MomentsOfInertia=[1 1 1]  MomentsOfInertiaUnits=kg*m^2  GraphicOpacity=1.0  ProductsOfInertia=[0 0 0]  ProductsOfInertiaUnits=kg*m^2  GraphicShininess=75  GraphicSpecularColor=[0.5 0.5 0.5 1.0]  GraphicVisPropType=SimpleVisualProperties
  Prismatic Joint1 : sm_lib/Joints/Prismatic Joint  JointMode=Normal  SenseConstraintForce=off  SenseConstraintForceX=off  SenseConstraintForceY=off  SenseConstraintForceZ=off  SenseConstraintTorque=off  SenseConstraintTorqueX=off  SenseConstraintTorqueY=off  SenseConstraintTorqueZ=off  SenseTotalForce=off  SenseTotalForceX=off  SenseTotalForceY=off  SenseTotalForceZ=off  SenseTotalTorque=off  SenseTotalTorqueX=off  SenseTotalTorqueY=off  SenseTotalTorqueZ=off  CompositeWrenchDir=FollowerOnBase  CompositeWrenchFrame=BaseFrame  EquilibriumPosition=0  EquilibriumPositionUnits=m  SpringStiffness=0  SpringStiffnessUnits=N/m  DampingCoefficient=b_c  DampingCoefficientUnits=N/(m/s)  TorqueActuationMode=InputTorque  MotionActuationMode=ComputedMotion  SensePosition=on  SenseVelocity=off  SenseAcceleration=off  SenseTorqueForce=off  SenseLowerLimitTorqueForce=off  SenseUpperLimitTorqueForce=off  LowerLimitSpecify=on  LowerLimitBound=-l_t/2  LowerLimitBoundUnits=m  LowerLimitStiffness=1e6  LowerLimitStiffnessUnits=N/m  LowerLimitDamping=1e3  LowerLimitDampingUnits=N/(m/s)  LowerLimitTransitionRegionWidth=1e-4  LowerLimitTransitionRegionWidthUnits=m  UpperLimitSpecify=on  UpperLimitBound=l_t/2  UpperLimitBoundUnits=m  UpperLimitStiffness=1e6  UpperLimitStiffnessUnits=N/m  UpperLimitDamping=1e3  UpperLimitDampingUnits=N/(m/s)  UpperLimitTransitionRegionWidth=1e-4  UpperLimitTransitionRegionWidthUnits=m  PositionTargetSpecify=off  PositionTargetPriority=High  PositionTargetValue=0  PositionTargetValueUnits=m  VelocityTargetSpecify=off  VelocityTargetPriority=High  VelocityTargetValue=0  VelocityTargetValueUnits=m/s
  Revolute Joint : sm_lib/Joints/Revolute Joint  JointMode=Normal  SenseConstraintForce=off  SenseConstraintForceX=off  SenseConstraintForceY=off  SenseConstraintForceZ=off  SenseConstraintTorque=off  SenseConstraintTorqueX=off  SenseConstraintTorqueY=off  SenseConstraintTorqueZ=off  SenseTotalForce=off  SenseTotalForceX=off  SenseTotalForceY=off  SenseTotalForceZ=off  SenseTotalTorque=off  SenseTotalTorqueX=off  SenseTotalTorqueY=off  SenseTotalTorqueZ=off  CompositeWrenchDir=FollowerOnBase  CompositeWrenchFrame=BaseFrame  EquilibriumPosition=0  EquilibriumPositionUnits=deg  SpringStiffness=0  SpringStiffnessUnits=N*m/deg  DampingCoefficient=b_p  DampingCoefficientUnits=N*m/(rad/s)  TorqueActuationMode=NoTorque  MotionActuationMode=ComputedMotion  SensePosition=on  SenseVelocity=off  SenseAcceleration=off  SenseTorqueForce=off  SenseLowerLimitTorqueForce=off  SenseUpperLimitTorqueForce=off  LowerLimitSpecify=off  LowerLimitBound=-90  LowerLimitBoundUnits=deg  LowerLimitStiffness=1e4  LowerLimitStiffnessUnits=N*m/deg  LowerLimitDamping=10  LowerLimitDampingUnits=N*m/(deg/s)  LowerLimitTransitionRegionWidth=0.1  LowerLimitTransitionRegionWidthUnits=deg  UpperLimitSpecify=off  UpperLimitBound=90  UpperLimitBoundUnits=deg  UpperLimitStiffness=1e4  UpperLimitStiffnessUnits=N*m/deg  UpperLimitDamping=10  UpperLimitDampingUnits=N*m/(deg/s)  UpperLimitTransitionRegionWidth=0.1  UpperLimitTransitionRegionWidthUnits=deg  PositionTargetSpecify=off  PositionTargetPriority=High  PositionTargetValue=0  PositionTargetValueUnits=deg  VelocityTargetSpecify=off  VelocityTargetPriority=High  VelocityTargetValue=0  VelocityTargetValueUnits=deg/s
  Rigid Transform : sm_lib/Frames and Transforms/Rigid Transform  TranslationMethod=None  TranslationStandardOffset=0  TranslationLengthUnit=m  TranslationStandardAxis=+Z  TranslationCartesianOffset=[0 0 0]  TranslationROffset=0  TranslationROffsetUnits=m  TranslationZOffset=0  TranslationZOffsetUnits=m  TranslationThetaOffset=0  TranslationThetaOffsetUnits=deg  RotationMethod=StandardAxis  RotationAngleUnits=deg  RotationStandardAxis=+Y  RotationAngle=90  RotationArbitraryAxis=[0 0 1]  FollAlignAxisA=+X  BaseAlignAxisA=+Y  FollAlignAxisB=+Y  BaseAlignAxisB=+Z  RotationSequenceAxes=FollowerAxes  RotationSequence=XYX  RotationSequenceAngles=[0 0 0]  RotationSequenceAnglesUnits=deg  RotationMatrix=[1 0 0; 0 1 0; 0 0 1]
  Rigid Transform1 : sm_lib/Frames and Transforms/Rigid Transform  TranslationMethod=None  TranslationStandardOffset=0  TranslationLengthUnit=m  TranslationStandardAxis=+Z  TranslationCartesianOffset=[0 0 0]  TranslationROffset=0  TranslationROffsetUnits=m  TranslationZOffset=0  TranslationZOffsetUnits=m  TranslationThetaOffset=0  TranslationThetaOffsetUnits=deg  RotationMethod=StandardAxis  RotationAngleUnits=deg  RotationStandardAxis=-Y  RotationAngle=90  RotationArbitraryAxis=[0 0 1]  FollAlignAxisA=+X  BaseAlignAxisA=+Y  FollAlignAxisB=+Y  BaseAlignAxisB=+Z  RotationSequenceAxes=FollowerAxes  RotationSequence=XYX  RotationSequenceAngles=[0 0 0]  RotationSequenceAnglesUnits=deg  RotationMatrix=[1 0 0; 0 1 0; 0 0 1]
  Rigid Transform2 : sm_lib/Frames and Transforms/Rigid Transform  TranslationMethod=None  TranslationStandardOffset=0  TranslationLengthUnit=m  TranslationStandardAxis=+Z  TranslationCartesianOffset=[0 0 0]  TranslationROffset=0  TranslationROffsetUnits=m  TranslationZOffset=0  TranslationZOffsetUnits=m  TranslationThetaOffset=0  TranslationThetaOffsetUnits=deg  RotationMethod=StandardAxis  RotationAngleUnits=deg  RotationStandardAxis=+X  RotationAngle=90  RotationArbitraryAxis=[0 0 1]  FollAlignAxisA=+X  BaseAlignAxisA=+Y  FollAlignAxisB=+Y  BaseAlignAxisB=+Z  RotationSequenceAxes=FollowerAxes  RotationSequence=XYX  RotationSequenceAngles=[0 0 0]  RotationSequenceAnglesUnits=deg  RotationMatrix=[1 0 0; 0 1 0; 0 0 1]
  Rigid Transform3 : sm_lib/Frames and Transforms/Rigid Transform  TranslationMethod=Cartesian  TranslationStandardOffset=0  TranslationLengthUnit=m  TranslationStandardAxis=+Z  TranslationCartesianOffset=[l_p 0 0]  TranslationROffset=0  TranslationROffsetUnits=m  TranslationZOffset=0  TranslationZOffsetUnits=m  TranslationThetaOffset=0  TranslationThetaOffsetUnits=deg  RotationMethod=StandardAxis  RotationAngleUnits=deg  RotationStandardAxis=-X  RotationAngle=90  RotationArbitraryAxis=[0 0 1]  FollAlignAxisA=+X  BaseAlignAxisA=+Y  FollAlignAxisB=+Y  BaseAlignAxisB=+Z  RotationSequenceAxes=FollowerAxes  RotationSequence=XYX  RotationSequenceAngles=[0 0 0]  RotationSequenceAnglesUnits=deg  RotationMatrix=[1 0 0; 0 1 0; 0 0 1]
  Rigid Transform4 : sm_lib/Frames and Transforms/Rigid Transform  TranslationMethod=None  TranslationStandardOffset=0  TranslationLengthUnit=m  TranslationStandardAxis=+Z  TranslationCartesianOffset=[0 0 0]  TranslationROffset=0  TranslationROffsetUnits=m  TranslationZOffset=0  TranslationZOffsetUnits=m  TranslationThetaOffset=0  TranslationThetaOffsetUnits=deg  RotationMethod=StandardAxis  RotationAngleUnits=deg  RotationStandardAxis=+Z  RotationAngle=90  RotationArbitraryAxis=[0 0 1]  FollAlignAxisA=+X  BaseAlignAxisA=+Y  FollAlignAxisB=+Y  BaseAlignAxisB=+Z  RotationSequenceAxes=FollowerAxes  RotationSequence=XYX  RotationSequenceAngles=[0 0 0]  RotationSequenceAnglesUnits=deg  RotationMatrix=[1 0 0; 0 1 0; 0 0 1]
  Rigid Transform5 : sm_lib/Frames and Transforms/Rigid Transform  TranslationMethod=Cartesian  TranslationStandardOffset=0  TranslationLengthUnit=m  TranslationStandardAxis=+Z  TranslationCartesianOffset=[l_p 0 0]  TranslationROffset=0  TranslationROffsetUnits=m  TranslationZOffset=0  TranslationZOffsetUnits=m  TranslationThetaOffset=0  TranslationThetaOffsetUnits=deg  RotationMethod=None  RotationAngleUnits=deg  RotationStandardAxis=-X  RotationAngle=90  RotationArbitraryAxis=[0 0 1]  FollAlignAxisA=+X  BaseAlignAxisA=+Y  FollAlignAxisB=+Y  BaseAlignAxisB=+Z  RotationSequenceAxes=FollowerAxes  RotationSequence=XYX  RotationSequenceAngles=[0 0 0]  RotationSequenceAnglesUnits=deg  RotationMatrix=[1 0 0; 0 1 0; 0 0 1]
  Simulink-PS Converter : nesl_utility/Simulink-PS Converter  PhysicalDomain=network_engine_domain  SubClassName=ps_input  LeftPortType=input  RightPortType=output  PseudoPeriodic=off  Frequencies=[]  NoiseDistribution=none  NoiseParameters=[]  Unit=1  AffineConversion=off  FilteringAndDerivatives=provide  SimscapeFilterOrder=1  InputFilterTimeConstant=0.001  UdotUserProvided=0
      settings: SourceProductBaseCode=PW,SS
  System : PMIOPort  Side=Left
  doAngle : PMIOPort  Port=2  Side=Left
  DoCartPosition : PMIOPort  Port=3  Side=Left
  wires:
  force/1 -> Simulink-PS Converter/1
  connections:
  Rigid Transform/LConn1 -- System/RConn1
  Rigid Transform1/RConn1 -- Rigid Transform2/LConn1 -- Brick Solid/RConn1
  Rigid Transform3/LConn1 -- Revolute Joint/RConn1
  Rigid Transform3/RConn1 -- Rigid Transform5/LConn1 -- Brick Solid1/RConn1
  Rigid Transform4/RConn1 -- Revolute Joint/LConn1
  Rigid Transform4/LConn1 -- Rigid Transform2/RConn1
  Brick Solid2/RConn1 -- Rigid Transform5/RConn1
  Revolute Joint/RConn2 -- doAngle/RConn1
  Prismatic Joint1/LConn1 -- Rigid Transform/RConn1
  Prismatic Joint1/RConn2 -- DoCartPosition/RConn1
  Prismatic Joint1/RConn1 -- Rigid Transform1/LConn1
  Simulink-PS Converter/RConn1 -- Prismatic Joint1/LConn2
